simulink model "Single_phase_inverter"  (R2022a)
settings: Solver=VariableStepAuto  StartTime=0.0  StopTime=PLECS_SIM_time  FixedStep=time_step  MaxStep=1e-4  RelTol=1e-3
undefined symbols (not defined in the file or in its folder): plecs
settings Model: Creator=kvkhh  LastModifiedBy=kvkhh
settings DataIOCC: ReturnWorkspaceOutputs=off
settings DebuggingCC: UnconnectedInputMsg=warning  UnconnectedOutputMsg=warning  UnconnectedLineMsg=warning
settings RTWCC: DLArmComputeVersion=19.05

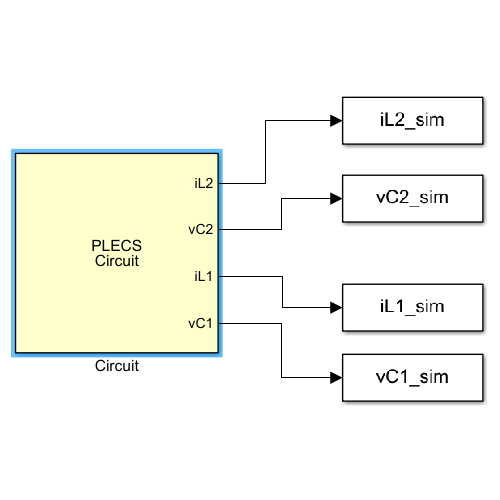
[thumbnail: Simulink's stored preview of the top-level diagram]
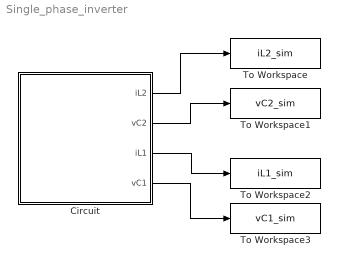
== system Single_phase_inverter ==
  Circuit : Subsystem  LoadFcn=plecs('sl', 200);  InitFcn=plecs('sl', 214);  StartFcn=plecs('sl', 208);  StopFcn=plecs('sl', 209);  mask(PlecsCircuit){PLECSData=<binary blob, 6300 chars, not shown>}
      mask prompts: PLECSData "PLECS Data (Do not delete or modify!)"
      mask init:
      | % PLACE CUSTOM INITIALIZATIONS ABOVE
      | % DO NOT REMOVE
      | plecs('sl', 215);
      | % DO NOT REMOVE
      settings: CopyFcn=plecs('sl', 203);  DeleteFcn=plecs('sl', 205);  UndoDeleteFcn=plecs('sl', 206);  PreSaveFcn=plecs('sl', 211);  PostSaveFcn=plecs('sl', 201);  NameChangeFcn=plecs('sl', 210);  DestroyFcn=plecs('sl', 207);  PreCopyFcn=plecs('sl', 216);  OpenFcn=plecs('sl', 202);  ErrorFcn=plerrorfcn
      mask Help: web(['file:///' fullfile(plecsdoc, 'creatingacircuit.html')])
      mask Display: disp('PLECS\nCircuit')
  To Workspace : ToWorkspace  VariableName=iL2_sim  SaveFormat=Structure With Time  SampleTime=-1
  To Workspace1 : ToWorkspace  VariableName=vC2_sim  SaveFormat=Structure With Time  SampleTime=-1
  To Workspace2 : ToWorkspace  VariableName=iL1_sim  SaveFormat=Structure With Time  SampleTime=-1
  To Workspace3 : ToWorkspace  VariableName=vC1_sim  SaveFormat=Structure With Time  SampleTime=-1
  wires:
  Circuit/1(iL2) -> To Workspace/1
  Circuit/2(vC2) -> To Workspace1/1
  Circuit/3(iL1) -> To Workspace2/1
  Circuit/4(vC1) -> To Workspace3/1

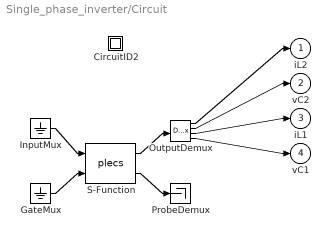
== system Single_phase_inverter/Circuit ==
  " CircuitID2 " : Subsystem
  " GateMux " : Ground
  " InputMux " : Ground
  " OutputDemux " : Demux  Outputs=[ 1 1 1 1 ]
  " ProbeDemux " : Terminator
  " S-Function " : S-Function  FunctionName=plecs  SFunctionDeploymentMode=off  EnableBusSupport=off
  iL2 : Outport  PortDimensions=1
  vC2 : Outport  Port=2  PortDimensions=1
  iL1 : Outport  Port=3  PortDimensions=1
  vC1 : Outport  Port=4  PortDimensions=1
  wires:
  " InputMux "/1 -> " S-Function "/1
  " GateMux "/1 -> " S-Function "/2
  " S-Function "/1 -> " OutputDemux "/1
  " S-Function "/2 -> " ProbeDemux "/1
  " OutputDemux "/1 -> iL2/1
  " OutputDemux "/2 -> vC2/1
  " OutputDemux "/3 -> iL1/1
  " OutputDemux "/4 -> vC1/1

== system Single_phase_inverter/Circuit/ CircuitID2  ==
